simulink model "buoyDetector"  (Simulink 7.6)
settings: Solver=FixedStepDiscrete  StartTime=0.0  StopTime=10.0  FixedStep=2  RelTol=1e-3
values from neighbouring files (symbols this model uses):
  Buoy_Max_Eccentricity = 1.2    [VisionConstants.m]
  Buoy_Max_Extent = 0.9    [VisionConstants.m]
  Buoy_Min_Extent = 0.1    [VisionConstants.m]
  Iter_Segment_Thresh = 60    [VisionConstants.m]
undefined symbols (not defined in the file or in its folder): jet, Rec, SDTV
libraries: vipconversions x4, vipgeotforms x3, vipsrcs x1, viptextngfix x1, vipsnks x1
settings Model: Creator=auvt  LastModifiedBy=auvt

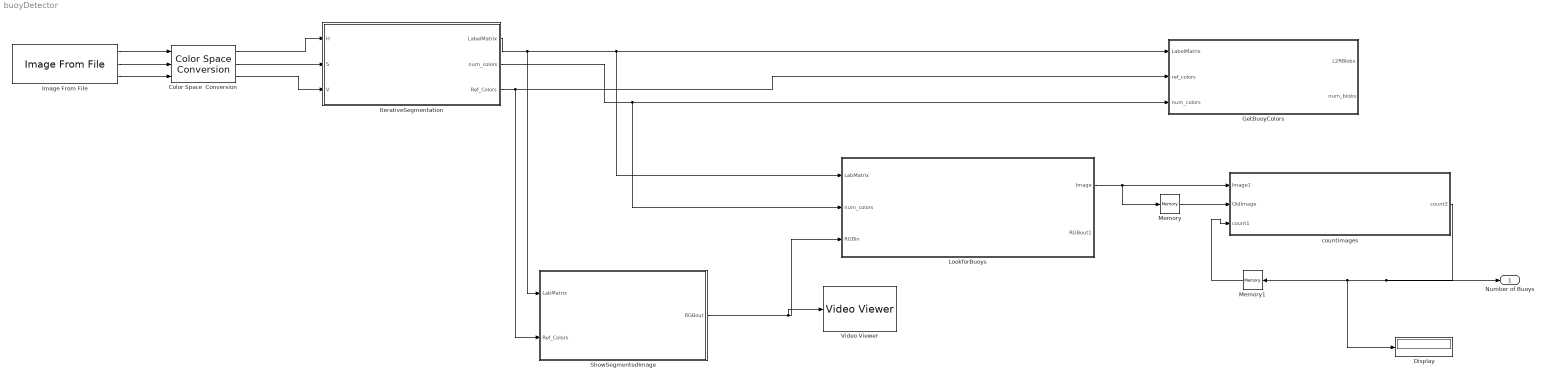
== system buoyDetector ==
  Color Space  Conversion : vipconversions/Color Space  Conversion  conversion=Obsolete  conversionActive=R'G'B' to HSV  wp_str=D65  rec=Rec. 601 (SDTV)  sys=1125/60/2:1  imagePorts=Separate color signals
  Display : Display
  GetBuoyColors : Subsystem
      settings: UndoDeleteFcn=Stateflow.SLINSF.SimulinkMan.restorePreDeleteFcn  PreDeleteFcn=Stateflow.SLINSF.SimulinkMan.removePreDeleteFcn
  Image From File : vipsrcs/Image From File  Tag=vipblks_nd  DialogController=vipDDGCreate  DialogControllerArgs=DataTag0  SystemSampleTime=-1  FileName=/home/auvt/testBuoys.png  imagePorts=Separate color signals  Ts=inf  ImageDataType=double  Signed=on  WordLength=16  sdImageDataType=uint(8)  FractionLengthMode=User-defined  FractionLength=15  OutPortLabels=R|G|B
  IterativeSegmentation : Subsystem
      settings: UndoDeleteFcn=Stateflow.SLINSF.SimulinkMan.restorePreDeleteFcn  PreDeleteFcn=Stateflow.SLINSF.SimulinkMan.removePreDeleteFcn
  LookforBuoys : Subsystem
      settings: UndoDeleteFcn=Stateflow.SLINSF.SimulinkMan.restorePreDeleteFcn  PreDeleteFcn=Stateflow.SLINSF.SimulinkMan.removePreDeleteFcn
  Memory : Memory
  Memory1 : Memory
  ShowSegmentedImage : Subsystem
      settings: UndoDeleteFcn=Stateflow.SLINSF.SimulinkMan.restorePreDeleteFcn  PreDeleteFcn=Stateflow.SLINSF.SimulinkMan.removePreDeleteFcn
  Video Viewer : vipsnks/Video Viewer  DialogControllerArgs=DataTag6  inputType=Obsolete7b  imagePorts=One multidimensional signal  useColorMap=off  colormapValue=jet(256)  specRange=off  minInputVal=0  maxInputVal=255  FigPos=[2707 511 410 300]  AxisZoom=on  trueSizedOnce=off  OpenAtMdlStart=on
  countimages : Stateflow chart  TreatAsAtomicUnit=on
  Number of Buoys : Outport
  wires:
  IterativeSegmentation/1(LabelMatrix) -> GetBuoyColors/1(LabelMatrix), LookforBuoys/1(LabMatrix), ShowSegmentedImage/1(LabMatrix)
  IterativeSegmentation/3(Ref_Colors) -> GetBuoyColors/2(ref_colors), ShowSegmentedImage/2(Ref_Colors)
  IterativeSegmentation/2(num_colors) -> GetBuoyColors/3(num_colors), LookforBuoys/2(num_colors)
  ShowSegmentedImage/1(RGBout) -> LookforBuoys/3(RGBin), Video Viewer/1
  LookforBuoys/1(Image) -> countimages/1(Image1), Memory/1
  Memory/1 -> countimages/2(OldImage)
  countimages/1(count2) -> Number of Buoys/1, Display/1, Memory1/1
  Color Space  Conversion/1 -> IterativeSegmentation/1(H)
  Color Space  Conversion/2 -> IterativeSegmentation/2(S)
  Color Space  Conversion/3 -> IterativeSegmentation/3(V)
  Memory1/1 -> countimages/3(count1)
  Image From File/1 -> Color Space  Conversion/1
  Image From File/2 -> Color Space  Conversion/2
  Image From File/3 -> Color Space  Conversion/3

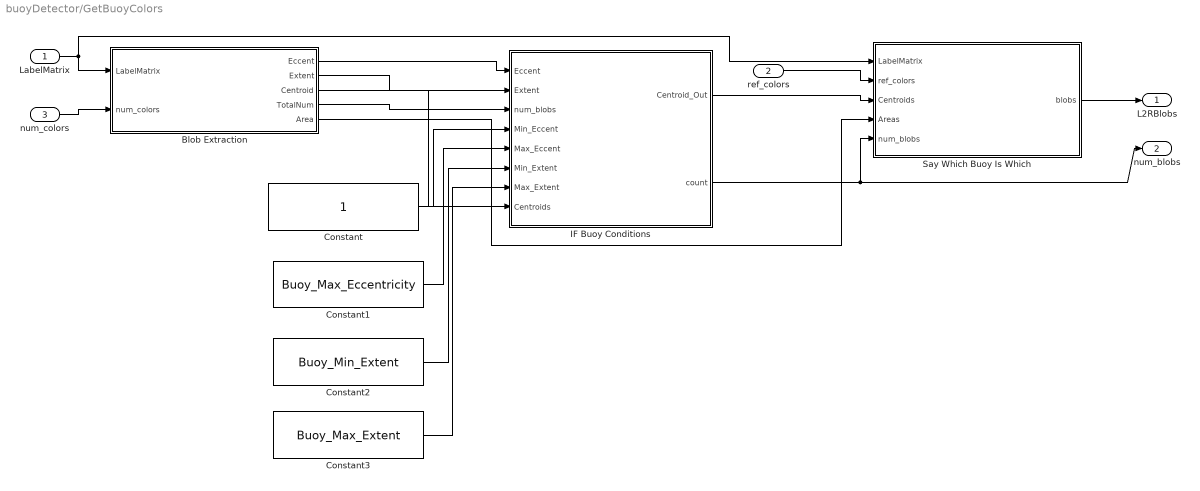
== system buoyDetector/GetBuoyColors ==
  LabelMatrix : Inport  PortDimensions=[120 160]
  ref_colors : Inport  Port=2  PortDimensions=[50 ,3]
  num_colors : Inport  Port=3
  Blob Extraction : Stateflow chart  TreatAsAtomicUnit=on
  Constant : Constant  SampleTime=-1
  Constant1 : Constant  Value=Buoy_Max_Eccentricity  SampleTime=-1
  Constant2 : Constant  Value=Buoy_Min_Extent  SampleTime=-1
  Constant3 : Constant  Value=Buoy_Max_Extent  SampleTime=-1
  IF Buoy Conditions : Stateflow chart  TreatAsAtomicUnit=on
  Say Which Buoy Is Which : Stateflow chart  TreatAsAtomicUnit=on
  L2RBlobs : Outport  PortDimensions=[50 4]
  num_blobs : Outport  Port=2
  wires:
  IF Buoy Conditions/2(count) -> num_blobs/1, Say Which Buoy Is Which/5(num_blobs)
  Blob Extraction/5(Area) -> Say Which Buoy Is Which/4(Areas)
  Say Which Buoy Is Which/1(blobs) -> L2RBlobs/1
  ref_colors/1 -> Say Which Buoy Is Which/2(ref_colors)
  IF Buoy Conditions/1(Centroid_Out) -> Say Which Buoy Is Which/3(Centroids)
  Blob Extraction/3(Centroid) -> IF Buoy Conditions/8(Centroids)
  Constant3/1 -> IF Buoy Conditions/7(Max_Extent)
  Constant2/1 -> IF Buoy Conditions/6(Min_Extent)
  Constant1/1 -> IF Buoy Conditions/5(Max_Eccent)
  Constant/1 -> IF Buoy Conditions/4(Min_Eccent)
  Blob Extraction/4(TotalNum) -> IF Buoy Conditions/3(num_blobs)
  Blob Extraction/2(Extent) -> IF Buoy Conditions/2(Extent)
  Blob Extraction/1(Eccent) -> IF Buoy Conditions/1(Eccent)
  num_colors/1 -> Blob Extraction/2(num_colors)
  LabelMatrix/1 -> Say Which Buoy Is Which/1(LabelMatrix), Blob Extraction/1(LabelMatrix)

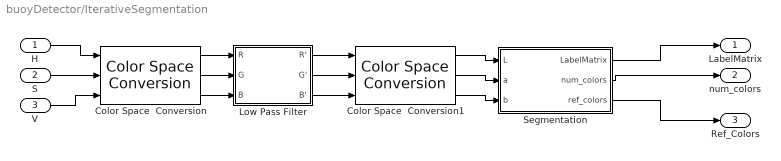
== system buoyDetector/IterativeSegmentation ==
  H : Inport  PortDimensions=[120 160]
  S : Inport  Port=2  PortDimensions=[120 160]
  V : Inport  Port=3  PortDimensions=[120 160]
  Color Space  Conversion : vipconversions/Color Space  Conversion  conversion=Obsolete  conversionActive=HSV to R'G'B'  wp_str=D50  rec=Rec. 601 (SDTV)  sys=1125/60/2:1  imagePorts=Separate color signals
  Color Space  Conversion1 : vipconversions/Color Space  Conversion  conversion=Obsolete  conversionActive=sR'G'B' to L*a*b*  wp_str=D50  rec=Rec. 601 (SDTV)  sys=1125/60/2:1  imagePorts=Separate color signals
  Low Pass Filter : Subsystem
  Segmentation : Subsystem
  LabelMatrix : Outport  PortDimensions=[120 160]
  num_colors : Outport  Port=2
  Ref_Colors : Outport  Port=3
  wires:
  Segmentation/3(ref_colors) -> Ref_Colors/1
  Segmentation/2(num_colors) -> num_colors/1
  Segmentation/1(LabelMatrix) -> LabelMatrix/1
  V/1 -> Color Space  Conversion/3
  S/1 -> Color Space  Conversion/2
  H/1 -> Color Space  Conversion/1
  Low Pass Filter/3(B') -> Color Space  Conversion1/3
  Low Pass Filter/2(G') -> Color Space  Conversion1/2
  Low Pass Filter/1(R') -> Color Space  Conversion1/1
  Color Space  Conversion1/3 -> Segmentation/3(b)
  Color Space  Conversion1/2 -> Segmentation/2(a)
  Color Space  Conversion1/1 -> Segmentation/1(L)
  Color Space  Conversion/3 -> Low Pass Filter/3(B)
  Color Space  Conversion/2 -> Low Pass Filter/2(G)
  Color Space  Conversion/1 -> Low Pass Filter/1(R)

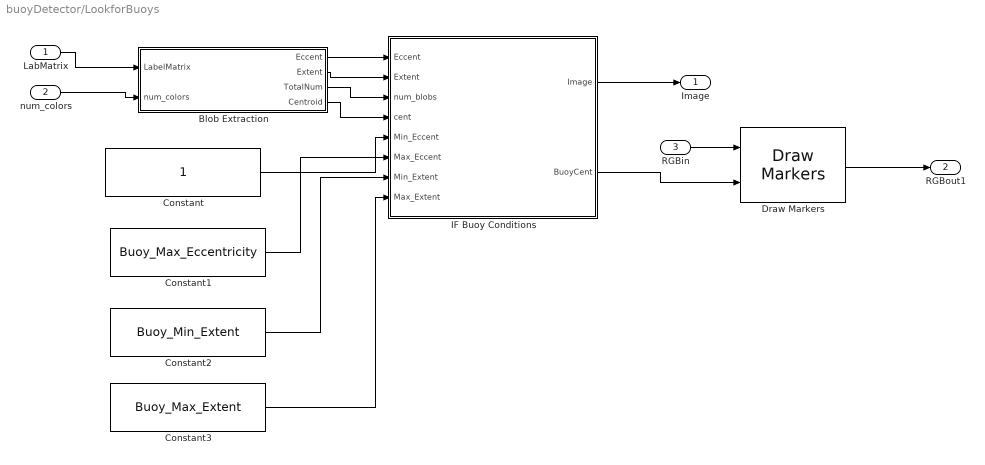
== system buoyDetector/LookforBuoys ==
  LabMatrix : Inport  PortDimensions=[120 160]
  num_colors : Inport  Port=2
  RGBin : Inport  Port=3  PortDimensions=[120 160 3]
  Blob Extraction : Stateflow chart  TreatAsAtomicUnit=on
  Constant : Constant  SampleTime=-1
  Constant1 : Constant  Value=Buoy_Max_Eccentricity  SampleTime=-1
  Constant2 : Constant  Value=Buoy_Min_Extent  SampleTime=-1
  Constant3 : Constant  Value=Buoy_Max_Extent  SampleTime=-1
  Draw Markers : viptextngfix/Draw Markers  DialogController=vipDDGCreate  DialogControllerArgs=DataTag4  shape=X-mark  size=7  fill=off  fillClrSource=Specify via dialog  display=User-specified value  intensity=200  color=[0 0 0]  opacity=0.6  viewport=Entire image  antialiasing=off  inType=Obsolete  imagePorts=One multidimensional signal  prodOutputMode=Binary point scaling  prodOutputWordLength=32  prodOutputFracLength=14  memoryMode=Specify word length  memoryWordLength=16  memoryFracLength=15  roundingMode=Floor  overflowMode=off
  IF Buoy Conditions : Stateflow chart  TreatAsAtomicUnit=on
  Image : Outport
  RGBout1 : Outport  Port=2  PortDimensions=[120 160 3]
  wires:
  Draw Markers/1 -> RGBout1/1
  RGBin/1 -> Draw Markers/1
  IF Buoy Conditions/2(BuoyCent) -> Draw Markers/2
  Blob Extraction/4(Centroid) -> IF Buoy Conditions/4(cent)
  Blob Extraction/3(TotalNum) -> IF Buoy Conditions/3(num_blobs)
  IF Buoy Conditions/1(Image) -> Image/1
  Constant3/1 -> IF Buoy Conditions/8(Max_Extent)
  Constant2/1 -> IF Buoy Conditions/7(Min_Extent)
  Constant1/1 -> IF Buoy Conditions/6(Max_Eccent)
  Constant/1 -> IF Buoy Conditions/5(Min_Eccent)
  Blob Extraction/2(Extent) -> IF Buoy Conditions/2(Extent)
  Blob Extraction/1(Eccent) -> IF Buoy Conditions/1(Eccent)
  num_colors/1 -> Blob Extraction/2(num_colors)
  LabMatrix/1 -> Blob Extraction/1(LabelMatrix)

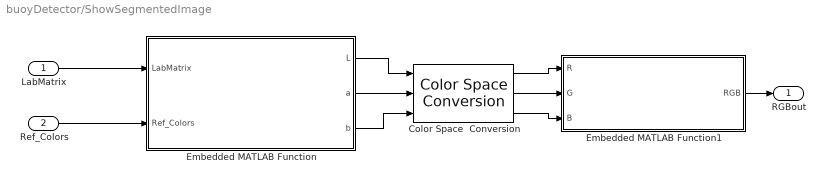
== system buoyDetector/ShowSegmentedImage ==
  LabMatrix : Inport  PortDimensions=[120 160]
  Ref_Colors : Inport  Port=2  PortDimensions=[50 3]
  Color Space  Conversion : vipconversions/Color Space  Conversion  conversion=Obsolete  conversionActive=L*a*b* to sR'G'B'  wp_str=D50  rec=Rec. 601 (SDTV)  sys=1125/60/2:1  imagePorts=Separate color signals
  Embedded MATLAB Function : Stateflow chart  TreatAsAtomicUnit=on
  Embedded MATLAB Function1 : Stateflow chart  TreatAsAtomicUnit=on
  RGBout : Outport  PortDimensions=[120 160 3]
  wires:
  Embedded MATLAB Function1/1(RGB) -> RGBout/1
  Color Space  Conversion/3 -> Embedded MATLAB Function1/3(B)
  Color Space  Conversion/2 -> Embedded MATLAB Function1/2(G)
  Color Space  Conversion/1 -> Embedded MATLAB Function1/1(R)
  Embedded MATLAB Function/3(b) -> Color Space  Conversion/3
  Embedded MATLAB Function/2(a) -> Color Space  Conversion/2
  Embedded MATLAB Function/1(L) -> Color Space  Conversion/1
  Ref_Colors/1 -> Embedded MATLAB Function/2(Ref_Colors)
  LabMatrix/1 -> Embedded MATLAB Function/1(LabMatrix)

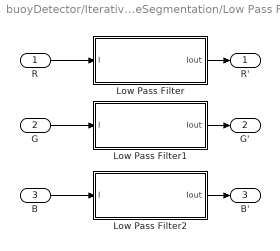
== system buoyDetector/IterativeSegmentation/Low Pass Filter ==
  R : Inport
  G : Inport  Port=2
  B : Inport  Port=3
  Low Pass Filter : Stateflow chart  TreatAsAtomicUnit=on
  Low Pass Filter1 : Stateflow chart  TreatAsAtomicUnit=on
  Low Pass Filter2 : Stateflow chart  TreatAsAtomicUnit=on
  R' : Outport
  G' : Outport  Port=2
  B' : Outport  Port=3
  wires:
  Low Pass Filter/1(Iout) -> R'/1
  Low Pass Filter2/1(Iout) -> B'/1
  Low Pass Filter1/1(Iout) -> G'/1
  B/1 -> Low Pass Filter2/1(I)
  G/1 -> Low Pass Filter1/1(I)
  R/1 -> Low Pass Filter/1(I)

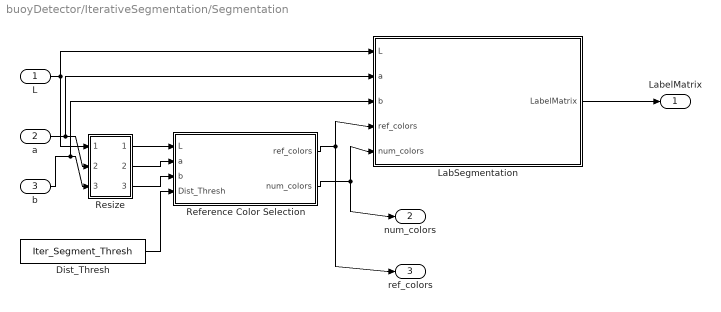
== system buoyDetector/IterativeSegmentation/Segmentation ==
  L : Inport
  a : Inport  Port=2
  b : Inport  Port=3
  Dist_Thresh : Constant  Value=Iter_Segment_Thresh  SampleTime=-1
  LabSegmentation : Stateflow chart  TreatAsAtomicUnit=on
  Reference Color Selection : Stateflow chart  TreatAsAtomicUnit=on
  Resize : Subsystem
  LabelMatrix : Outport
  num_colors : Outport  Port=2
  ref_colors : Outport  Port=3
  wires:
  Dist_Thresh/1 -> Reference Color Selection/4(Dist_Thresh)
  LabSegmentation/1(LabelMatrix) -> LabelMatrix/1
  Reference Color Selection/2(num_colors) -> num_colors/1, LabSegmentation/5(num_colors)
  Reference Color Selection/1(ref_colors) -> ref_colors/1, LabSegmentation/4(ref_colors)
  Resize/3(Out3) -> Reference Color Selection/3(b)
  Resize/2(Out2) -> Reference Color Selection/2(a)
  Resize/1(Out1) -> Reference Color Selection/1(L)
  b/1 -> LabSegmentation/3(b), Resize/3(In3)
  a/1 -> LabSegmentation/2(a), Resize/2(In2)
  L/1 -> LabSegmentation/1(L), Resize/1(In1)

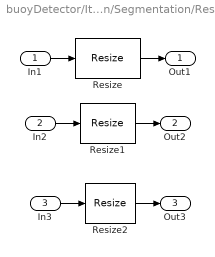
== system buoyDetector/IterativeSegmentation/Segmentation/Resize ==
  In1 : Inport
  In2 : Inport  Port=2
  In3 : Inport  Port=3
  Resize : vipgeotforms/Resize  DialogController=vipDDGCreate  DialogControllerArgs=DataTag1  specify=Number of output rows and columns  rfactor=[]  outCols=25  outRows=25  outRowsCols=[60 80]  interp_method=Bilinear  antialias=on  useROI=off  roiFlag=off  prodOutputMode=Binary point scaling  prodOutputWordLength=32  prodOutputFracLength=10  roundingMode=Nearest  overflowMode=on
  Resize1 : vipgeotforms/Resize  DialogController=vipDDGCreate  DialogControllerArgs=DataTag2  specify=Number of output rows and columns  rfactor=[200 150]  outCols=25  outRows=25  outRowsCols=[60 80]  interp_method=Bilinear  antialias=on  useROI=off  roiFlag=off  prodOutputMode=Binary point scaling  prodOutputWordLength=32  prodOutputFracLength=10  roundingMode=Nearest  overflowMode=on
  Resize2 : vipgeotforms/Resize  DialogController=vipDDGCreate  DialogControllerArgs=DataTag3  specify=Number of output rows and columns  rfactor=[200 150]  outCols=25  outRows=25  outRowsCols=[60 80]  interp_method=Bilinear  antialias=on  useROI=off  roiFlag=off  prodOutputMode=Binary point scaling  prodOutputWordLength=32  prodOutputFracLength=10  roundingMode=Nearest  overflowMode=on
  Out1 : Outport
  Out2 : Outport  Port=2
  Out3 : Outport  Port=3
  wires:
  Resize2/1 -> Out3/1
  In3/1 -> Resize2/1
  Resize1/1 -> Out2/1
  In2/1 -> Resize1/1
  Resize/1 -> Out1/1
  In1/1 -> Resize/1

== matlab function ShowSegmentedImage/Embedded MATLAB Function ==
  data: LabMatrix input double; L output double; Ref_Colors input double; a output double; b output double
function [L,a,b]=CombineSegmentedImage(LabMatrix,Ref_Colors)
% This function puts together the segmented imaged such that it can be shown

[rows, cols] = size(LabMatrix);
L = zeros(rows,cols);
a = zeros(rows,cols);
b = zeros(rows,cols);

for i = 1:rows
    for j = 1:cols
        L(i,j) = Ref_Colors(LabMatrix(i,j),1);
        a(i,j) = Ref_Colors(LabMatrix(i,j),2);
        b(i,j) = Ref_Colors(LabMatrix(i,j),3);
    end
end

return

== matlab function ShowSegmentedImage/Embedded MATLAB Function1 ==
  data: R input double; RGB output double; G input double; B input double
function RGB = SeparatetoSingleSignals(R,G,B)
% This function combines the separate color signals into a single 3-D signal

[rows, cols] = size(R);

RGB = zeros(rows,cols,3);

for i = 1:rows
    for j = 1:cols
        RGB(i,j,1) = R(i,j);
        RGB(i,j,2) = G(i,j);
        RGB(i,j,3) = B(i,j);
    end
end

return

== matlab function LookforBuoys/Blob Extraction ==
  data: LabelMatrix input double; Eccent output double; num_colors input double; Extent output double; TotalNum output double; Centroid output double
function [Eccent,Extent,TotalNum,Centroid] = GetBlobInfo(LabelMatrix, num_colors)
% This function will determine the characteristics of the blobs in an image
% given a label matrix defining the different binary images contained in a
% that label matrix

[rows, cols] = size(LabelMatrix);
LogicMatrix = false(rows,cols);

max_num_blobs = 50;
min_blob_area = 5;

Centroid = zeros(max_num_blobs,2);
Eccent = zeros(1,max_num_blobs);
Extent = zeros(1,max_num_blobs);

TotalNum = uint8(0);

persistent hblob
if isempty(hblob)
    hblob = video.BlobAnalysis('AreaOutputPort',false,'BoundingBoxOutputPort',false,...
        'CentroidOutputPort',true,'EccentricityOutputPort',true,'ExtentOutputPort',true,...
        'NumBlobsOutputPort',true,'MinimumBlobAreaSource','Property',...
        'MinimumBlobArea', min_blob_area);
end

for k = 1:num_colors
    for i = 1:rows
        for j = 1:cols
            if(LabelMatrix(i,j) ~= k)
                LogicMatrix(i,j) = false;
            else
                LogicMatrix(i,j) = true;
            end
        end
    end
    [TCentroid,TEccent,TExtent,TNumBlobs] = step(hblob,LogicMatrix);
    
    if(TotalNum+TNumBlobs < max_num_blobs)
        for i = 1:TNumBlobs
            Centroid(TotalNum+i,1) = TCentroid(1,i);
            Centroid(TotalNum+i,2) = TCentroid(2,i);
            Eccent(TotalNum+i) = TEccent(i);
            Extent(TotalNum+i) = TExtent(i);
        end
        TotalNum = TotalNum + TNumBlobs;
    end
end

return

== matlab function LookforBuoys/IF Buoy Conditions ==
  data: Eccent input double; Image output double; Extent input double; num_blobs input double; cent input double; Min_Eccent input double; Max_Eccent input double; Min_Extent input double; Max_Extent input double; BuoyCent output double
function [Image,BuoyCent] = BuoyConditions(Eccent,Extent,num_blobs, cent,Min_Eccent, Max_Eccent,Min_Extent,Max_Extent)
% This function will take in 2 1x10 vectors, eccent and extent to determine
% if there is a buoy present in the current image

Image = 0;
count = 0;
BuoyCent = ones(2,50);

for i = 1:num_blobs
    if((Eccent(i)>Min_Eccent) && (Eccent(i)<Max_Eccent) && (Extent(i)>Min_Extent) && (Extent(i)<Max_Extent))
        count = count + 1;
        BuoyCent(1,count) = cent(i,1);
        BuoyCent(2,count) = cent(i,2);
    end
end

if(count >= 3)
    Image = 1;
end

return

== matlab function GetBuoyColors/Blob Extraction ==
  data: LabelMatrix input double; Eccent output double; num_colors input double; Extent output double; Centroid output double; TotalNum output double; Area output double
function [Eccent,Extent,Centroid,TotalNum,Area] = GetBlobInfo(LabelMatrix, num_colors)
% This function will determine the characteristics of the blobs in an image
% given a label matrix defining the different binary images contained in a
% that label matrix

[rows, cols] = size(LabelMatrix);
LogicMatrix = false(rows,cols);

max_num_blobs = 50;
min_blob_area = 10;

Area = zeros(1,max_num_blobs);
Centroid = zeros(max_num_blobs,2);
Eccent = zeros(1,max_num_blobs);
Extent = zeros(1,max_num_blobs);

TotalNum = uint8(0);

persistent hblob
if isempty(hblob)
    hblob = video.BlobAnalysis('AreaOutputPort',true,'BoundingBoxOutputPort',false,...
        'CentroidOutputPort',true,'EccentricityOutputPort',true,'ExtentOutputPort',true,...
        'NumBlobsOutputPort',true,'MinimumBlobAreaSource','Property',...
        'MinimumBlobArea', min_blob_area);
end

for k = 1:num_colors
    for i = 1:rows
        for j = 1:cols
            if(LabelMatrix(i,j) ~= k)
                LogicMatrix(i,j) = false;
            else
                LogicMatrix(i,j) = true;
            end
        end
    end
    [TArea, TCentroid,TEccent,TExtent,TNumBlobs] = step(hblob,LogicMatrix);
    
    if(TNumBlobs+TotalNum < max_num_blobs)
        for i = 1:TNumBlobs
            Area(TotalNum+i) = TArea(i);
            Centroid(TotalNum+i,1) = TCentroid(1,i);
            Centroid(TotalNum+i,2) = TCentroid(2,i);
            Eccent(TotalNum+i) = TEccent(i);
            Extent(TotalNum+i) = TExtent(i);
        end
        TotalNum = TotalNum + TNumBlobs;
    end
end

return

== matlab function GetBuoyColors/IF Buoy Conditions ==
  data: Eccent input double; Centroid_Out output double; Extent input double; num_blobs input double; Min_Eccent input double; Max_Eccent input double; Min_Extent input double; Max_Extent input double; Centroids input double; count output double
function [Centroid_Out, count] = BuoyConditions(Eccent,Extent,num_blobs,Min_Eccent, Max_Eccent,Min_Extent,Max_Extent,Centroids)
% This function will take in 2 1x10 vectors, eccent and extent to determine
% the cenroids of the most circular objects in the image

count = 0;
Centroid_Out = zeros(50,2);


for i = 1:num_blobs
    if((Eccent(i)>Min_Eccent) && (Eccent(i)<Max_Eccent) && (Extent(i)>Min_Extent) && (Extent(i)<Max_Extent))
        count = count + 1;
        Centroid_Out(count,1) = Centroids(i,1);
        Centroid_Out(count,2) = Centroids(i,2);
    end
end

return

== matlab function GetBuoyColors/Say Which Buoy Is Which ==
  data: LabelMatrix input double; blobs output double; ref_colors input double; Centroids input double; Areas input double; num_blobs input double
function blobs  = WhichBuoyIsWhich(LabelMatrix,ref_colors,Centroids,Areas, num_blobs)
% This function determines which buoy is in which location, left, middle,
% or right.

max_num_blobs = 50;
colors = zeros(max_num_blobs,3);
centX = zeros(1,max_num_blobs);
centY = zeros(1,max_num_blobs);
reference = zeros(1,1);
blobs = zeros(max_num_blobs,4);

for i = 1:num_blobs
    centX(i) = floor(Centroids(i,2));
    centY(i) = floor(Centroids(i,1));
    if(centX(i) < 1)
        centX(i) = 1;
    end
    if(centY(i) < 1)
        centY(i) = 1;
    end
    
    reference = LabelMatrix(centY(i),centX(i));
    
    colors(i,1:3) = [ref_colors(reference,1), ref_colors(reference,2), ref_colors(reference,3)];
end

% Putting blobs in order from left to right
for i = 1:num_blobs
    [value ref] = min(centX);
    blobs(i,1) = colors(ref,1);
    blobs(i,2) = colors(ref,2);
    blobs(i,3) = colors(ref,3);
    blobs(i,4) = Areas(ref);
    centX(ref) = 1000;
end

return

== matlab function countimages ==
  data: Image1 input double; count2 output double; OldImage input double; count1 input double
function count2 = countimages(Image1, OldImage, count1)
% This function acts to count the number of consecutive times a particular
% image is recognized by the recognition software

count2 = count1;
if(Image1 == 1)
    count2 = count2 + 1;
else
    count2 = 0;
end

== matlab function IterativeSegmentation/Low Pass Filter/Low Pass Filter ==
  data: I input double; Iout output double
function Iout = GaussianBlurr(I)
% This function calculates the gaussian blur of an intensity image

sigma = sqrt(2);

Grows = 3;    % Gaussian matrix rows
Gcols = 3;    % Gaussian matrix columns

[Irows Icols] = size(I);

Iout = single(zeros(Irows,Icols));

Trows = Irows - Grows + 1;
Tcols = Icols - Gcols + 1;
Itemp = single(zeros(Trows,Tcols));

G = zeros(Grows,Gcols);

FirstRow = ceil(-Grows/2);
LastRow = floor(Grows/2);
FirstCol = ceil(-Gcols/2);
LastCol = floor(Gcols/2);
Gsum = 0;
for i=FirstRow:LastRow
    for j = FirstCol:LastCol
        G(i-FirstRow+1,j-FirstCol+1) = exp(-(j*j+i*i)/(2*sigma*sigma));
        Gsum = Gsum + G(i-FirstRow+1,j-FirstCol+1);
    end
end

G = G./Gsum;

Itemp = conv2(single(I),single(G),'valid');

% reflect boundaries to keep image the same size
% top
Iout((1:LastRow),(LastCol+1:Icols-LastCol)) = Itemp((1:LastRow),(1:Tcols));
% bottom
Iout((Irows-LastRow+1:Irows),(LastCol+1:Icols-LastCol)) = Itemp((Trows-LastRow+1:Trows),(1:Tcols));
% left
Iout((1+LastRow:Irows-LastRow),(1:LastCol)) = Itemp((1:Trows),(1:LastCol));
% right
Iout((1+LastRow:Irows-LastRow),(Icols-LastCol+1:Icols)) = Itemp((1:Trows),(Tcols-LastCol+1:Tcols));
% center
Iout((1+LastRow:Irows-LastRow),(1+LastCol:Icols-LastCol)) = Itemp;
% top left corner
Iout(1:LastRow,1:LastCol) = Itemp(1:LastRow,1:LastCol);
% top right corner
Iout(1:LastRow,Icols-LastCol:Icols) = Itemp(1:LastRow,Tcols-LastCol:Tcols);
% bottom left corner
Iout(Irows-LastRow:Irows,1:LastCol) = Itemp(Trows-LastRow:Trows,1:LastCol);
% bottom right corner
Iout(Irows-LastRow:Irows,Icols-LastCol:Icols) = Itemp(Trows-LastRow:Trows,Tcols-LastCol:Tcols);

return

== matlab function IterativeSegmentation/Low Pass Filter/Low Pass Filter1 ==
  data: I input double; Iout output double
function Iout = GaussianBlurr(I)
% This function calculates the gaussian blur of an intensity image

sigma = sqrt(2);

Grows = 3;    % Gaussian matrix rows
Gcols = 3;    % Gaussian matrix columns

[Irows Icols] = size(I);

Iout = single(zeros(Irows,Icols));

Trows = Irows - Grows + 1;
Tcols = Icols - Gcols + 1;
Itemp = single(zeros(Trows,Tcols));

G = zeros(Grows,Gcols);

FirstRow = ceil(-Grows/2);
LastRow = floor(Grows/2);
FirstCol = ceil(-Gcols/2);
LastCol = floor(Gcols/2);
Gsum = 0;
for i=FirstRow:LastRow
    for j = FirstCol:LastCol
        G(i-FirstRow+1,j-FirstCol+1) = exp(-(j*j+i*i)/(2*sigma*sigma));
        Gsum = Gsum + G(i-FirstRow+1,j-FirstCol+1);
    end
end

G = G./Gsum;

Itemp = conv2(single(I),single(G),'valid');

% reflect boundaries to keep image the same size
% top
Iout((1:LastRow),(LastCol+1:Icols-LastCol)) = Itemp((1:LastRow),(1:Tcols));
% bottom
Iout((Irows-LastRow+1:Irows),(LastCol+1:Icols-LastCol)) = Itemp((Trows-LastRow+1:Trows),(1:Tcols));
% left
Iout((1+LastRow:Irows-LastRow),(1:LastCol)) = Itemp((1:Trows),(1:LastCol));
% right
Iout((1+LastRow:Irows-LastRow),(Icols-LastCol+1:Icols)) = Itemp((1:Trows),(Tcols-LastCol+1:Tcols));
% center
Iout((1+LastRow:Irows-LastRow),(1+LastCol:Icols-LastCol)) = Itemp;
% top left corner
Iout(1:LastRow,1:LastCol) = Itemp(1:LastRow,1:LastCol);
% top right corner
Iout(1:LastRow,Icols-LastCol:Icols) = Itemp(1:LastRow,Tcols-LastCol:Tcols);
% bottom left corner
Iout(Irows-LastRow:Irows,1:LastCol) = Itemp(Trows-LastRow:Trows,1:LastCol);
% bottom right corner
Iout(Irows-LastRow:Irows,Icols-LastCol:Icols) = Itemp(Trows-LastRow:Trows,Tcols-LastCol:Tcols);

return

== matlab function IterativeSegmentation/Low Pass Filter/Low Pass Filter2 ==
  data: I input double; Iout output double
function Iout = GaussianBlurr(I)
% This function calculates the gaussian blur of an intensity image

sigma = sqrt(2);

Grows = 3;    % Gaussian matrix rows
Gcols = 3;    % Gaussian matrix columns

[Irows Icols] = size(I);

Iout = single(zeros(Irows,Icols));

Trows = Irows - Grows + 1;
Tcols = Icols - Gcols + 1;
Itemp = single(zeros(Trows,Tcols));

G = zeros(Grows,Gcols);

FirstRow = ceil(-Grows/2);
LastRow = floor(Grows/2);
FirstCol = ceil(-Gcols/2);
LastCol = floor(Gcols/2);
Gsum = 0;
for i=FirstRow:LastRow
    for j = FirstCol:LastCol
        G(i-FirstRow+1,j-FirstCol+1) = exp(-(j*j+i*i)/(2*sigma*sigma));
        Gsum = Gsum + G(i-FirstRow+1,j-FirstCol+1);
    end
end

G = G./Gsum;

Itemp = conv2(single(I),single(G),'valid');

% reflect boundaries to keep image the same size
% top
Iout((1:LastRow),(LastCol+1:Icols-LastCol)) = Itemp((1:LastRow),(1:Tcols));
% bottom
Iout((Irows-LastRow+1:Irows),(LastCol+1:Icols-LastCol)) = Itemp((Trows-LastRow+1:Trows),(1:Tcols));
% left
Iout((1+LastRow:Irows-LastRow),(1:LastCol)) = Itemp((1:Trows),(1:LastCol));
% right
Iout((1+LastRow:Irows-LastRow),(Icols-LastCol+1:Icols)) = Itemp((1:Trows),(Tcols-LastCol+1:Tcols));
% center
Iout((1+LastRow:Irows-LastRow),(1+LastCol:Icols-LastCol)) = Itemp;
% top left corner
Iout(1:LastRow,1:LastCol) = Itemp(1:LastRow,1:LastCol);
% top right corner
Iout(1:LastRow,Icols-LastCol:Icols) = Itemp(1:LastRow,Tcols-LastCol:Tcols);
% bottom left corner
Iout(Irows-LastRow:Irows,1:LastCol) = Itemp(Trows-LastRow:Trows,1:LastCol);
% bottom right corner
Iout(Irows-LastRow:Irows,Icols-LastCol:Icols) = Itemp(Trows-LastRow:Trows,Tcols-LastCol:Tcols);

return

== matlab function IterativeSegmentation/Segmentation/LabSegmentation ==
  data: L input double; LabelMatrix output double; a input double; b input double; ref_colors input double; num_colors input double
function LabelMatrix  = LabSegmentation(L,a,b,ref_colors,num_colors)
% This function generates the label matrix

[rows cols] = size(L);

Lout = zeros(rows,cols);
aout = zeros(rows,cols);
bout = zeros(rows,cols);

LabelMatrix = zeros(rows,cols);

for i = 1:rows
    for j = 1:cols
        min_dist = 1000;
        index = 1;
        for k = 1:num_colors
            dist = sqrt((ref_colors(k,1) - L(i,j))^2 + (ref_colors(k,2) - a(i,j))^2 + (ref_colors(k,3) - b(i,j))^2);
            if(dist < min_dist)
                min_dist = double(dist);
                index = k;
            end
        end
        LabelMatrix(i,j) = index;
    end
end

for i = 1:rows
    for j = 1:cols
        Lout(i,j) = ref_colors(LabelMatrix(i,j),1);
        aout(i,j) = ref_colors(LabelMatrix(i,j),2);
        bout(i,j) = ref_colors(LabelMatrix(i,j),3);
    end
end

cow = 1;

return

== matlab function IterativeSegmentation/Segmentation/Reference Color Selection ==
  data: L input double; ref_colors output double; a input double; b input double; num_colors output double; Dist_Thresh input double
function [ref_colors, num_colors] = Segmentation(L,a,b,Dist_Thresh)
% This function tries segmentation by adding new reference colors everytime
% a pixel is found with a distance greater than a certain amount from
% every other reference color

[rows cols] = size(L);

Dist_Threshold = Dist_Thresh;% L = 0 to 100, a = -100 to 100, b = -100 to 100
                    % max dist = 300 -> 60/300 is 20%
x = 1;  % coefficients determining distance calculation
y = 1.5;
z = 1.5;

max_num_colors = 50;
ref_colors = zeros(max_num_colors,3);   % At most 50 different reference colors
LabelMatrix = zeros(rows,cols);
num_colors = 1;

center_row = floor(rows/2);
center_col = floor(cols/2);

ref_colors(1,:) = [L(center_row,center_col) a(center_row,center_col) b(center_row,center_col)];

flag = 0;
i = 1;
j = 1;
while(i <= rows)        % perform initial segmentation
    while(i <= rows && flag == 0)
        while(j <= cols && flag == 0)
            k = 1;
            min_dist = 1000;
            index = 1;
            while(k <= num_colors)
                dist = sqrt(x*(ref_colors(k,1) - L(i,j))^2 + y*(ref_colors(k,2) - a(i,j))^2 + z*(ref_colors(k,3) - b(i,j))^2);
                if(min_dist > dist)
                    min_dist = double(dist);
                    index = k;
                end
                k = k + 1;
            end
            if(j == 117)
                cow = 1;
            end
            if(min_dist > Dist_Threshold && num_colors < max_num_colors)
                ref_colors(num_colors+1,:) = [L(i,j) a(i,j) b(i,j)];
                num_colors = num_colors + 1;
                flag = 1;
                i = 0;
                j = 0;
            else
                LabelMatrix(i,j) = index;
            end
            j = j + 1;
        end
        j = 1;
        i = i + 1;
    end
    flag = 0;
end

% Go through image once more to get more accurate values for the different regions
ref_color_L_avg = zeros(50,1);
ref_color_a_avg = zeros(50,1);
ref_color_b_avg = zeros(50,1);
color_count = zeros(50,1);
for i = 1:rows
    for j = 1:cols
        index = LabelMatrix(i,j);
        ref_color_L_avg(index) = ref_color_L_avg(index) + L(i,j);
        ref_color_a_avg(index) = ref_color_a_avg(index) + a(i,j);
        ref_color_b_avg(index) = ref_color_b_avg(index) + b(i,j);
        color_count(index) = color_count(index) + 1;
    end
end
ref_color_L_avg = ref_color_L_avg ./ color_count;
ref_color_a_avg = ref_color_a_avg ./ color_count;
ref_color_b_avg = ref_color_b_avg ./ color_count;

for i = 1:num_colors
    ref_colors(i,1) = ref_color_L_avg(i);
    ref_colors(i,2) = ref_color_a_avg(i);
    ref_colors(i,3) = ref_color_b_avg(i);
end

return
